simulink model "ProyectoIntegrador2025"  (R2024b)
settings: Solver=VariableStepAuto  StartTime=0.0  StopTime=80  FixedStep=0.1  RelTol=1e-3
values from neighbouring files (symbols this model uses):
  A = Lm / I    (= 19.8203592814)    [Grafico_comparacion_controlador_continuo_discreto.m]    (also in Grafico_comparacion_modelo_linealizado.m = -C * sin(theta_eq) / I; PIDf_Asignacion_Polos.m; SimulacionModelosMallaCerradaConControlador.m; Variables_sistema_para_simulink.m)
  angulo_equilibrio = 10 * (pi/180)    (= 0.174532925199)    [Grafico_comparacion_controlador_continuo_discreto.m]    (also in Obtener_modelo_motor.m = 0; PIDf_Asignacion_Polos.m = 0; SimulacionModelosMallaCerradaConControlador.m = i * (pi/180); Variables_sistema_para_simulink.m = 0)
  B = C * sin(angulo_equilibrio) / I    [Grafico_comparacion_controlador_continuo_discreto.m]    (also in Grafico_comparacion_modelo_linealizado.m = 19.8203592814; PIDf_Asignacion_Polos.m; SimulacionModelosMallaCerradaConControlador.m; Variables_sistema_para_simulink.m)
  C = Pcp * Lcp + Pv1 * Lv1 - Pc * Lc - Pv2 * Lv2 - Pj * Lj - Pm * Lm    (= -0.1326097161)    [Constantes_helicoptero.m]    (also in Grafica_PWMvsFuerza_equilibrio.m = -0.1326; Grafica_validacion_superpuestas.m = -0.1326; Grafico_comparacion_controlador_continuo_discreto.m = -0.1326; Grafico_comparacion_modelo_linealizado.m = -0.1326)
  condicion_inicial_angulo_modelo_no_lineal = angulo_equilibrio    (= 0.174532925199)    [Grafico_comparacion_controlador_continuo_discreto.m]    (also in SimulacionModelosMallaCerradaConControlador.m = angulo_equilibrio)
  fuerza_equilibrio = -(C * cos(angulo_equilibrio)) / Lm    [Grafico_comparacion_controlador_continuo_discreto.m]    (also in SimulacionModelosMallaCerradaConControlador.m)
  I = Icp + Im + Ij + Iv1 + Iv2 + Ic    (= 0.0166790788666)    [Constantes_helicoptero.m]    (also in Grafica_PWMvsFuerza_equilibrio.m = 0.0167; Grafica_validacion_superpuestas.m = 0.0167; Grafico_comparacion_controlador_continuo_discreto.m = 0.0167; Grafico_comparacion_modelo_linealizado.m = 0.0167)
  Kd = 102.99198    [Grafico_comparacion_controlador_continuo_discreto.m]    (also in PIDf_Asignacion_Polos.m = (alpha2 - B - Kp*m*A)/(alpha1*m*A); SimulacionModelosMallaCerradaConControlador.m; test.m = 57.0171)
  Ki = 95.63817    [Grafico_comparacion_controlador_continuo_discreto.m]    (also in PIDf_Asignacion_Polos.m = (alpha4)/(alpha1*m*A); SimulacionModelosMallaCerradaConControlador.m; test.m = 0.5088)
  Kp = 106.62644    [Grafico_comparacion_controlador_continuo_discreto.m]    (also in PIDf_Asignacion_Polos.m = (alpha3-alpha1*B-(alpha4/alpha1))/(alpha1*m*A); SimulacionModelosMallaCerradaConControlador.m; test.m = 10.8703)
  Lm = 2 * Lv2 + 0.014    (= 0.331)    [Constantes_helicoptero.m]    (also in Grafica_PWMvsFuerza_equilibrio.m; Grafica_validacion_superpuestas.m = 0.35; Grafico_comparacion_controlador_continuo_discreto.m; Grafico_comparacion_modelo_linealizado.m)
  m = 0.001586    [Grafica_PWMvsFuerza_equilibrio.m]    (also in Grafico_comparacion_controlador_continuo_discreto.m; Obtener_modelo_motor.m = coeficientes(1); PIDf_Asignacion_Polos.m; SimulacionModelosMallaCerradaConControlador.m)
  N = 12.00000    (= 12)    [Grafico_comparacion_controlador_continuo_discreto.m]    (also in PIDf_Asignacion_Polos.m = alpha1; SimulacionModelosMallaCerradaConControlador.m; test.m = 5.4539)
  PWM_equilibrio = (fuerza_equilibrio-r)/m    [Grafico_comparacion_controlador_continuo_discreto.m]    (also in SimulacionModelosMallaCerradaConControlador.m = (fuerza_equilibrio - r) / m)
  r = -1.597768    [Grafica_PWMvsFuerza_equilibrio.m]    (also in Grafico_comparacion_controlador_continuo_discreto.m = -1.692631; Obtener_modelo_motor.m = coeficientes(2); SimulacionModelosMallaCerradaConControlador.m)
  ref = 0    [Grafico_comparacion_controlador_continuo_discreto.m]    (also in PIDf_Asignacion_Polos.m = 1; SimulacionModelosMallaCerradaConControlador.m = angulo_equilibrio)
libraries: slpidlib x3
settings Model: Creator=UTEC-5695  LastModifiedBy=lucas

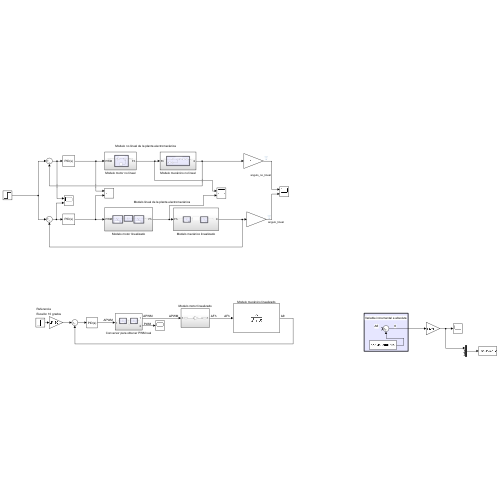
[thumbnail: Simulink's stored preview of the top-level diagram]
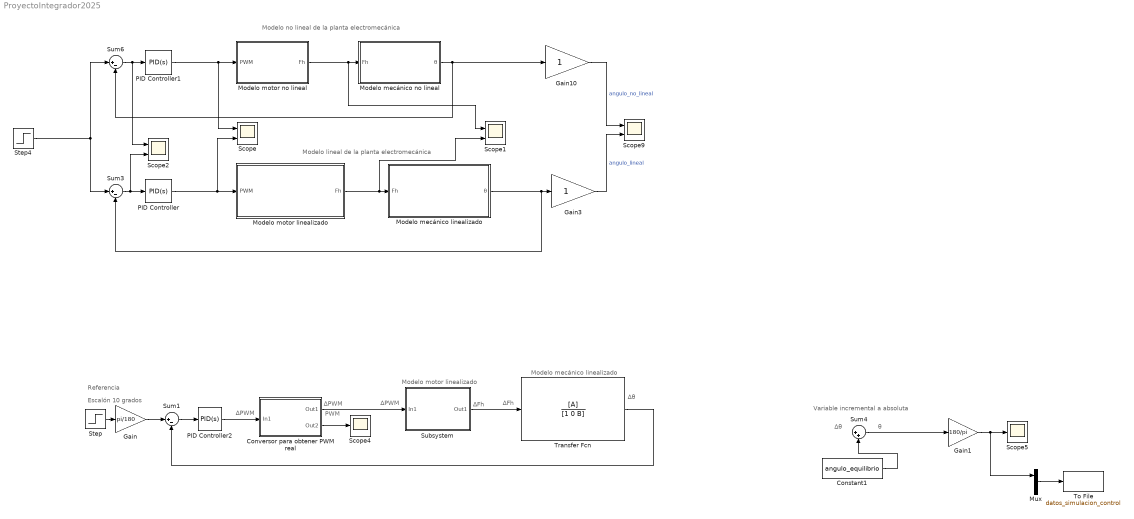
== system ProyectoIntegrador2025 ==
  note: Referencia
  note: Escalón 10 grados
  note: PWM
  note: Modelo no lineal de la planta electromecánica
  note: Modelo lineal de la planta electromecánica
  note: Modelo motor linealizado
  note: Δθ
  note: ΔFh
  note: Modelo mecánico linealizado
  note: ΔPWM
  note: ΔPWM
  note: ΔPWM
  note: ΔFh
  note: Δθ
  note: θ
  note: Variable incremental a absoluta
  Constant1 : Constant  Value=angulo_equilibrio
  Conversor para obtener PWM real : Subsystem
  Gain : Gain  Gain=pi/180
  Gain1 : Gain  Gain=180/pi
  Gain10 : Gain
  Gain3 : Gain
  Modelo mecánico linealizado : Subsystem
  Modelo mecánico no lineal : Subsystem
  Modelo motor linealizado : Subsystem
  Modelo motor no lineal : Subsystem
  Mux : Mux  Inputs=3
  PID Controller : slpidlib/PID Controller  Controller=PID  Form=Parallel  TimeDomain=Continuous-time  UseExternalTs=off  SampleTime=-1  IntegratorMethod=Forward Euler  FilterMethod=Forward Euler  ControllerParametersSource=internal  P=93.8725143926059  I=17.4427346666791  UseKiTs=off  D=124.052527033934  UseExternalDerivativeSource=off  N=21.6474087647294  UseFilter=on  TunerSelectOption=Transfer Function Based (PID Tuner App)  InitialConditionSource=internal  InitialConditionForIntegrator=0  InitialConditionForFilter=0  DifferentiatorICPrevScaledInput=0  ExternalReset=none  TrackingMode=off  Kt=1  LimitOutput=off  SatLimitsSource=internal  UpperSaturationLimit=inf  LowerSaturationLimit=-inf  LinearizeAsGain=on  AntiWindupMode=none  Kb=1  LimitIntegrator=off  UpperIntegratorSaturationLimit=inf  LowerIntegratorSaturationLimit=-inf  POutMin=[]  POutMax=[]  IOutMin=[]  IOutMax=[]  DOutMin=[]  DOutMax=[]  NOutMin=[]  NOutMax=[]  SumOutMin=[]  SumOutMax=[]  SaturationOutMin=[]  SaturationOutMax=[]  PParamMin=[]  PParamMax=[]  IParamMin=[]  IParamMax=[]  DParamMin=[]  DParamMax=[]  NParamMin=[]  NParamMax=[]  KbParamMin=[]  KbParamMax=[]  KtParamMin=[]  KtParamMax=[]  KbOutMin=[]  KbOutMax=[]  KtOutMin=[]  KtOutMax=[]  IntegratorOutMin=[]  IntegratorOutMax=[]  FilterOutMin=[]  FilterOutMax=[]  SumI1OutMin=[]  SumI1OutMax=[]  SumI2OutMin=[]  SumI2OutMax=[]  SumI3OutMin=[]  SumI3OutMax=[]  SumI4OutMin=[]  SumI4OutMax=[]  SumDOutMin=[]  SumDOutMax=[]  DifferentiatorOutMin=[]  DifferentiatorOutMax=[]  FilterDiffOutCoefMin=[]  FilterDiffOutCoefMax=[]  ReciprocalOutMin=[]  ReciprocalOutMax=[]  SumDenOutMin=[]  SumDenOutMax=[]  SumNumOutMin=[]  SumNumOutMax=[]  DivideOutMin=[]  DivideOutMax=[]  UdiffTsProdOutMin=[]  UdiffTsProdOutMax=[]  NTsProdOutMin=[]  NTsProdOutMax=[]  UintegralTsProdOutMin=[]  UintegralTsProdOutMax=[]  UngainTsProdOutMin=[]  UngainTsProdOutMax=[]  ClampingZeroOutDataTypeStr=Inherit: Inherit via back propagation  ClampingZeroOutMin=[]  ClampingZeroOutMax=[]  FilterDenConstantOutDataTypeStr=Inherit: Inherit via back propagation  FilterDenConstantOutMin=[]  FilterDenConstantOutMax=[]  PCopyOutDataTypeStr=Inherit: Inherit via back propagation  PCopyOutMin=[]  PCopyOutMax=[]  NCopyOutDataTypeStr=Inherit: Inherit via back propagation  NCopyOutMin=[]  NCopyOutMax=[]  IntegratorContinuousStateAttributes=''  IntegratorStateMustResolveToSignalObject=off  IntegratorRTWStateStorageClass=Auto  FilterContinuousStateAttributes=''  FilterStateMustResolveToSignalObject=off  FilterRTWStateStorageClass=Auto  ParallelPVariant=InternalParameters  IdealPVariant=Disabled  IVariant=InternalParameters  DVariant=InternalParameters  IntegratorVariant=Continuous  SatVariant=Disabled  AWVariant=Passthrough  PCopyVariant=Disabled  TRVariant=Disabled  FdbkBlocksVariant=Forward  IdealPFdbkVariant=Disabled  SatFdbkVariant=Disabled  DerivativeFilterVariant=ContFilter  NVariant=InternalParameters  NCopyVariant=Disabled  FilterICVariant=InternalICsFilter  IntegratorICVariant=InternalICs  ExternalResetVariant=Disabled  TRSumVariant=Passthrough  SumFdbkVariant=Disabled  SumVariant=Sum_PID  TsampFilterVariant=InternalTs  TsampNgainVariant=Passthrough  TsampIntegralVariant=Disabled_SignalSpec  ExternalSaturationOutDataTypeStr=Inherit: Same as second input  DerivativeSourceVariant=ErrorSignal  PreIntVariant=InternalPreInt
  PID Controller1 : slpidlib/PID Controller  Controller=PID  Form=Parallel  TimeDomain=Continuous-time  UseExternalTs=off  SampleTime=-1  IntegratorMethod=Forward Euler  FilterMethod=Forward Euler  ControllerParametersSource=internal  P=Kp  I=Ki  UseKiTs=off  D=Kd  UseExternalDerivativeSource=off  N=N  UseFilter=on  TunerSelectOption=Transfer Function Based (PID Tuner App)  InitialConditionSource=internal  InitialConditionForIntegrator=0  InitialConditionForFilter=1  DifferentiatorICPrevScaledInput=0  ExternalReset=none  TrackingMode=off  Kt=1  LimitOutput=off  SatLimitsSource=internal  UpperSaturationLimit=inf  LowerSaturationLimit=-inf  LinearizeAsGain=on  AntiWindupMode=none  Kb=1  LimitIntegrator=off  UpperIntegratorSaturationLimit=inf  LowerIntegratorSaturationLimit=-inf  POutMin=[]  POutMax=[]  IOutMin=[]  IOutMax=[]  DOutMin=[]  DOutMax=[]  NOutMin=[]  NOutMax=[]  SumOutMin=[]  SumOutMax=[]  SaturationOutMin=[]  SaturationOutMax=[]  PParamMin=[]  PParamMax=[]  IParamMin=[]  IParamMax=[]  DParamMin=[]  DParamMax=[]  NParamMin=[]  NParamMax=[]  KbParamMin=[]  KbParamMax=[]  KtParamMin=[]  KtParamMax=[]  KbOutMin=[]  KbOutMax=[]  KtOutMin=[]  KtOutMax=[]  IntegratorOutMin=[]  IntegratorOutMax=[]  FilterOutMin=[]  FilterOutMax=[]  SumI1OutMin=[]  SumI1OutMax=[]  SumI2OutMin=[]  SumI2OutMax=[]  SumI3OutMin=[]  SumI3OutMax=[]  SumI4OutMin=[]  SumI4OutMax=[]  SumDOutMin=[]  SumDOutMax=[]  DifferentiatorOutMin=[]  DifferentiatorOutMax=[]  FilterDiffOutCoefMin=[]  FilterDiffOutCoefMax=[]  ReciprocalOutMin=[]  ReciprocalOutMax=[]  SumDenOutMin=[]  SumDenOutMax=[]  SumNumOutMin=[]  SumNumOutMax=[]  DivideOutMin=[]  DivideOutMax=[]  UdiffTsProdOutMin=[]  UdiffTsProdOutMax=[]  NTsProdOutMin=[]  NTsProdOutMax=[]  UintegralTsProdOutMin=[]  UintegralTsProdOutMax=[]  UngainTsProdOutMin=[]  UngainTsProdOutMax=[]  ClampingZeroOutDataTypeStr=Inherit: Inherit via back propagation  ClampingZeroOutMin=[]  ClampingZeroOutMax=[]  FilterDenConstantOutDataTypeStr=Inherit: Inherit via back propagation  FilterDenConstantOutMin=[]  FilterDenConstantOutMax=[]  PCopyOutDataTypeStr=Inherit: Inherit via back propagation  PCopyOutMin=[]  PCopyOutMax=[]  NCopyOutDataTypeStr=Inherit: Inherit via back propagation  NCopyOutMin=[]  NCopyOutMax=[]  IntegratorContinuousStateAttributes=''  IntegratorStateMustResolveToSignalObject=off  IntegratorRTWStateStorageClass=Auto  FilterContinuousStateAttributes=''  FilterStateMustResolveToSignalObject=off  FilterRTWStateStorageClass=Auto  ParallelPVariant=InternalParameters  IdealPVariant=Disabled  IVariant=InternalParameters  DVariant=InternalParameters  IntegratorVariant=Continuous  SatVariant=Disabled  AWVariant=Passthrough  PCopyVariant=Disabled  TRVariant=Disabled  FdbkBlocksVariant=Forward  IdealPFdbkVariant=Disabled  SatFdbkVariant=Disabled  DerivativeFilterVariant=ContFilter  NVariant=InternalParameters  NCopyVariant=Disabled  FilterICVariant=InternalICsFilter  IntegratorICVariant=InternalICs  ExternalResetVariant=Disabled  TRSumVariant=Passthrough  SumFdbkVariant=Disabled  SumVariant=Sum_PID  TsampFilterVariant=InternalTs  TsampNgainVariant=Passthrough  TsampIntegralVariant=Disabled_SignalSpec  ExternalSaturationOutDataTypeStr=Inherit: Same as second input  DerivativeSourceVariant=ErrorSignal  PreIntVariant=InternalPreInt
  PID Controller2 : slpidlib/PID Controller  Controller=PID  Form=Parallel  TimeDomain=Continuous-time  UseExternalTs=off  SampleTime=-1  IntegratorMethod=Forward Euler  FilterMethod=Forward Euler  ControllerParametersSource=internal  P=Kp  I=Ki  UseKiTs=off  D=Kd  UseExternalDerivativeSource=off  N=N  UseFilter=on  TunerSelectOption=Transfer Function Based (PID Tuner App)  InitialConditionSource=internal  InitialConditionForIntegrator=0  InitialConditionForFilter=0  DifferentiatorICPrevScaledInput=0  ExternalReset=none  TrackingMode=off  Kt=1  LimitOutput=off  SatLimitsSource=internal  UpperSaturationLimit=inf  LowerSaturationLimit=-inf  LinearizeAsGain=on  AntiWindupMode=none  Kb=1  LimitIntegrator=off  UpperIntegratorSaturationLimit=inf  LowerIntegratorSaturationLimit=-inf  POutMin=[]  POutMax=[]  IOutMin=[]  IOutMax=[]  DOutMin=[]  DOutMax=[]  NOutMin=[]  NOutMax=[]  SumOutMin=[]  SumOutMax=[]  SaturationOutMin=[]  SaturationOutMax=[]  PParamMin=[]  PParamMax=[]  IParamMin=[]  IParamMax=[]  DParamMin=[]  DParamMax=[]  NParamMin=[]  NParamMax=[]  KbParamMin=[]  KbParamMax=[]  KtParamMin=[]  KtParamMax=[]  KbOutMin=[]  KbOutMax=[]  KtOutMin=[]  KtOutMax=[]  IntegratorOutMin=[]  IntegratorOutMax=[]  FilterOutMin=[]  FilterOutMax=[]  SumI1OutMin=[]  SumI1OutMax=[]  SumI2OutMin=[]  SumI2OutMax=[]  SumI3OutMin=[]  SumI3OutMax=[]  SumI4OutMin=[]  SumI4OutMax=[]  SumDOutMin=[]  SumDOutMax=[]  DifferentiatorOutMin=[]  DifferentiatorOutMax=[]  FilterDiffOutCoefMin=[]  FilterDiffOutCoefMax=[]  ReciprocalOutMin=[]  ReciprocalOutMax=[]  SumDenOutMin=[]  SumDenOutMax=[]  SumNumOutMin=[]  SumNumOutMax=[]  DivideOutMin=[]  DivideOutMax=[]  UdiffTsProdOutMin=[]  UdiffTsProdOutMax=[]  NTsProdOutMin=[]  NTsProdOutMax=[]  UintegralTsProdOutMin=[]  UintegralTsProdOutMax=[]  UngainTsProdOutMin=[]  UngainTsProdOutMax=[]  ClampingZeroOutDataTypeStr=Inherit: Inherit via back propagation  ClampingZeroOutMin=[]  ClampingZeroOutMax=[]  FilterDenConstantOutDataTypeStr=Inherit: Inherit via back propagation  FilterDenConstantOutMin=[]  FilterDenConstantOutMax=[]  PCopyOutDataTypeStr=Inherit: Inherit via back propagation  PCopyOutMin=[]  PCopyOutMax=[]  NCopyOutDataTypeStr=Inherit: Inherit via back propagation  NCopyOutMin=[]  NCopyOutMax=[]  IntegratorContinuousStateAttributes=''  IntegratorStateMustResolveToSignalObject=off  IntegratorRTWStateStorageClass=Auto  FilterContinuousStateAttributes=''  FilterStateMustResolveToSignalObject=off  FilterRTWStateStorageClass=Auto  ParallelPVariant=InternalParameters  IdealPVariant=Disabled  IVariant=InternalParameters  DVariant=InternalParameters  IntegratorVariant=Continuous  SatVariant=Disabled  AWVariant=Passthrough  PCopyVariant=Disabled  TRVariant=Disabled  FdbkBlocksVariant=Forward  IdealPFdbkVariant=Disabled  SatFdbkVariant=Disabled  DerivativeFilterVariant=ContFilter  NVariant=InternalParameters  NCopyVariant=Disabled  FilterICVariant=InternalICsFilter  IntegratorICVariant=InternalICs  ExternalResetVariant=Disabled  TRSumVariant=Passthrough  SumFdbkVariant=Disabled  SumVariant=Sum_PID  TsampFilterVariant=InternalTs  TsampNgainVariant=Passthrough  TsampIntegralVariant=Disabled_SignalSpec  ExternalSaturationOutDataTypeStr=Inherit: Same as second input  DerivativeSourceVariant=ErrorSignal  PreIntVariant=InternalPreInt
  Scope{,1..2,9} (4 alike) : Scope  NumInputPorts=2
  Scope4 : Scope
  Scope5 : Scope
  Step : Step  Time=0  After=10  SampleTime=0
  Step4 : Step  Time=0  After=ref  SampleTime=0
  Subsystem : Subsystem
  Sum1 : Sum  Inputs=|+-
  Sum3 : Sum  Inputs=|+-
  Sum4 : Sum  Inputs=|++
  Sum6 : Sum  Inputs=|+-
  To File : ToFile  Filename=datos_simulacion_control  SaveFormat=Timeseries
  Transfer Fcn : TransferFcn  Numerator=[A]  Denominator=[1 0 B]
  wires:
  Sum6/1 -> Scope2/1, PID Controller1/1
  Step4/1 -> Sum3/1, Sum6/1
  Gain10/1 -> Scope9/1  "angulo_no_lineal"
  Gain3/1 -> Scope9/2  "angulo_lineal"
  Sum3/1 -> Scope2/2, PID Controller/1
  Modelo mecánico linealizado/1(θ) -> Gain3/1, Sum3/2
  Modelo mecánico no lineal/1(θ) -> Gain10/1, Sum6/2
  Modelo motor linealizado/1(Fh) -> Scope1/2, Modelo mecánico linealizado/1(Fh)
  Modelo motor no lineal/1(Fh) -> Scope1/1, Modelo mecánico no lineal/1(Fh)
  PID Controller1/1 -> Scope/1, Modelo motor no lineal/1(PWM)
  PID Controller/1 -> Scope/2, Modelo motor linealizado/1(PWM)
  PID Controller2/1 -> Conversor para obtener PWM real/1(In1)
  Sum1/1 -> PID Controller2/1
  Step/1 -> Gain/1
  Conversor para obtener PWM real/2(Out2) -> Scope4/1
  Conversor para obtener PWM real/1(Out1) -> Subsystem/1(In1)
  Subsystem/1(Out1) -> Transfer Fcn/1
  Constant1/1 -> Sum4/2
  Sum4/1 -> Gain1/1
  Transfer Fcn/1 -> Sum1/2
  Gain/1 -> Sum1/1
  Gain1/1 -> Mux/1, Scope5/1
  Mux/1 -> To File/1

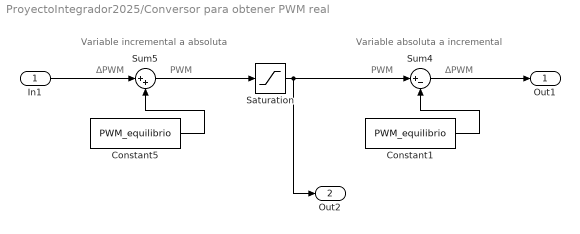
== system ProyectoIntegrador2025/Conversor para obtener PWM real ==
  note: Variable incremental a absoluta
  note: ΔPWM
  note: PWM
  note: ΔPWM
  note: Variable absoluta a incremental
  note: PWM
  In1 : Inport
  Constant1 : Constant  Value=PWM_equilibrio
  Constant5 : Constant  Value=PWM_equilibrio
  Saturation : Saturate  UpperLimit=2000  LowerLimit=1000
  Sum4 : Sum  Inputs=|+-
  Sum5 : Sum  Inputs=|++
  Out1 : Outport
  Out2 : Outport  Port=2
  wires:
  Constant5/1 -> Sum5/2
  Sum5/1 -> Saturation/1
  Constant1/1 -> Sum4/2
  Sum4/1 -> Out1/1
  In1/1 -> Sum5/1
  Saturation/1 -> Sum4/1, Out2/1

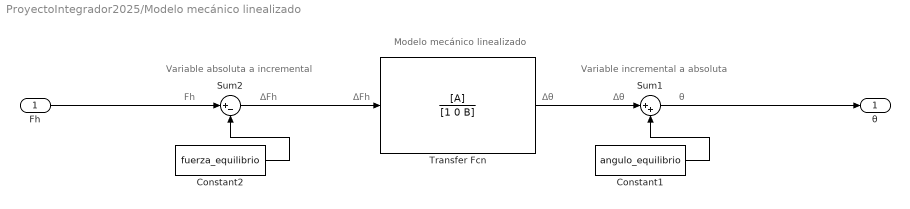
== system ProyectoIntegrador2025/Modelo mecánico linealizado ==
  note: Modelo mecánico linealizado
  note: Variable incremental a absoluta
  note: Fh
  note: Variable absoluta a incremental
  note: ΔFh
  note: Δθ
  note: θ
  note: Δθ
  note: ΔFh
  Fh : Inport
  Constant1 : Constant  Value=angulo_equilibrio
  Constant2 : Constant  Value=fuerza_equilibrio
  Sum1 : Sum  Inputs=|++
  Sum2 : Sum  Inputs=|+-
  Transfer Fcn : TransferFcn  Numerator=[A]  Denominator=[1 0 B]
  θ : Outport
  wires:
  Constant1/1 -> Sum1/2
  Constant2/1 -> Sum2/2
  Transfer Fcn/1 -> Sum1/1
  Fh/1 -> Sum2/1
  Sum2/1 -> Transfer Fcn/1
  Sum1/1 -> θ/1

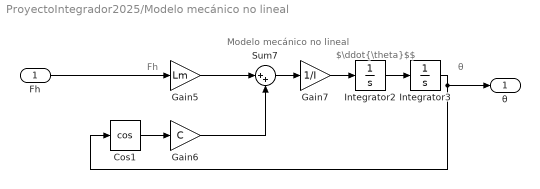
== system ProyectoIntegrador2025/Modelo mecánico no lineal ==
  note: θ
  note: Modelo mecánico no lineal
  note: Fh
  note: $\ddot{\theta}$$
  Fh : Inport
  Cos1 : Trigonometry  Operator=cos
  Gain5 : Gain  Gain=Lm
  Gain6 : Gain  Gain=C
  Gain7 : Gain  Gain=1/I
  Integrator2 : Integrator
  Integrator3 : Integrator  InitialCondition=condicion_inicial_angulo_modelo_no_lineal
  Sum7 : Sum  Inputs=|++
  θ : Outport
  wires:
  Integrator3/1 -> θ/1, Cos1/1
  Gain6/1 -> Sum7/2
  Cos1/1 -> Gain6/1
  Fh/1 -> Gain5/1
  Gain7/1 -> Integrator2/1
  Sum7/1 -> Gain7/1
  Gain5/1 -> Sum7/1
  Integrator2/1 -> Integrator3/1

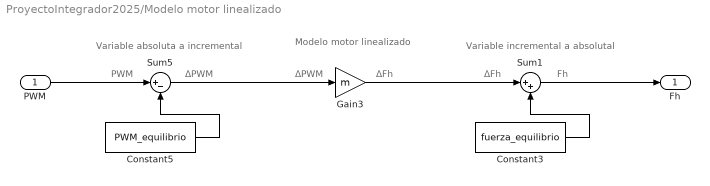
== system ProyectoIntegrador2025/Modelo motor linealizado ==
  note: PWM
  note: Variable absoluta a incremental
  note: ΔPWM
  note: ΔFh
  note: Fh
  note: Modelo motor linealizado
  note: Variable incremental a absolutal
  note: ΔFh
  note: ΔPWM
  PWM : Inport
  Constant3 : Constant  Value=fuerza_equilibrio
  Constant5 : Constant  Value=PWM_equilibrio
  Gain3 : Gain  Gain=m
  Sum1 : Sum  Inputs=|++
  Sum5 : Sum  Inputs=|+-
  Fh : Outport
  wires:
  Sum5/1 -> Gain3/1
  PWM/1 -> Sum5/1
  Sum1/1 -> Fh/1
  Constant5/1 -> Sum5/2
  Gain3/1 -> Sum1/1
  Constant3/1 -> Sum1/2

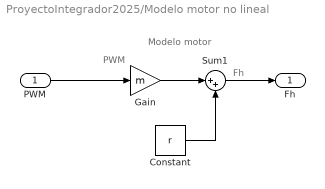
== system ProyectoIntegrador2025/Modelo motor no lineal ==
  note: PWM
  note: Fh
  note: Modelo motor
  PWM : Inport
  Constant : Constant  Value=r
  Gain : Gain  Gain=m
  Sum1 : Sum  Inputs=|++
  Fh : Outport
  wires:
  Constant/1 -> Sum1/2
  Gain/1 -> Sum1/1
  Sum1/1 -> Fh/1
  PWM/1 -> Gain/1

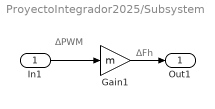
== system ProyectoIntegrador2025/Subsystem ==
  note: ΔPWM
  note: ΔFh
  In1 : Inport
  Gain1 : Gain  Gain=m
  Out1 : Outport
  wires:
  Gain1/1 -> Out1/1
  In1/1 -> Gain1/1
